simulink model "Appl_PaComfort_CtrlModel"  (R2018b)
settings: configuration reference "CodeConfig_10_ms" (kept outside this file)
undefined symbols (not defined in the file): D_CLOSE, D_InitDelayTime, D_OPEN, D_SoftDistancePaLegnth, D_WelcomeDistance, FALSE, TRUE
libraries: DareLib x44, simulink x1
(part 1 of 2)
settings Model: Creator=Administrator  LastModifiedBy=Administrator
settings ConfigSetRef: SourceLocation=Base Workspace

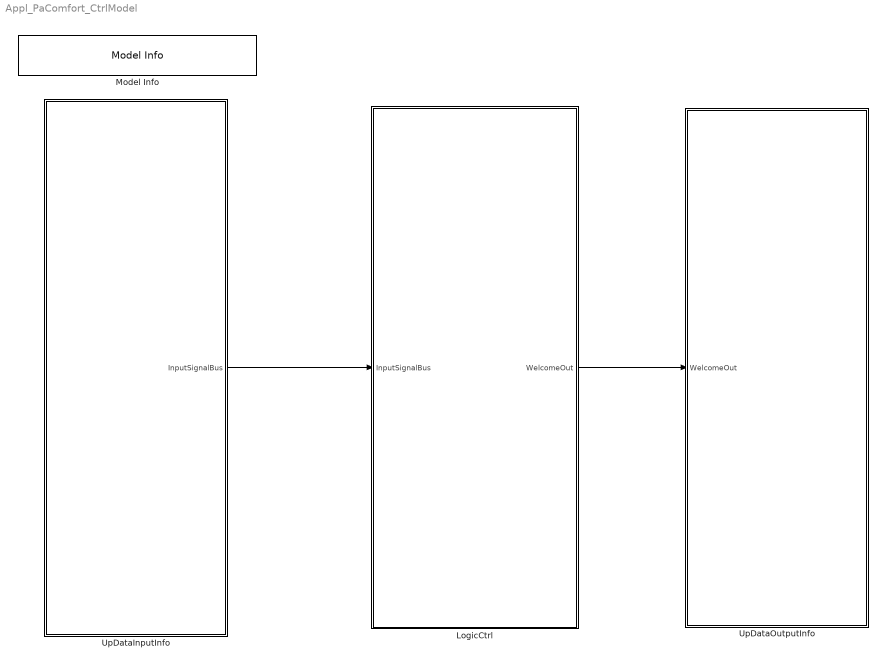
== system Appl_PaComfort_CtrlModel ==
  LogicCtrl : Subsystem  Priority=2  TreatAsAtomicUnit=on
      settings: RTWSystemCode=Nonreusable function  RTWFcnNameOpts=Use subsystem name
  Model Info : simulink/Model-Wide Utilities/Model Info  Frame=on  DisplayStringWithTags=Version：%<ModelVersion>  HorizontalTextAlignment=Center  LeftAlignmentValue=0.5
  UpDataInputInfo : Subsystem  Priority=1  TreatAsAtomicUnit=on
      settings: RTWSystemCode=Nonreusable function  RTWFcnNameOpts=Use subsystem name
  UpDataOutputInfo : Subsystem  Priority=3  TreatAsAtomicUnit=on
      settings: RTWSystemCode=Nonreusable function  RTWFcnNameOpts=Use subsystem name
  wires:
  LogicCtrl/1(WelcomeOut) -> UpDataOutputInfo/1(WelcomeOut)
  UpDataInputInfo/1(InputSignalBus) -> LogicCtrl/1(InputSignalBus)

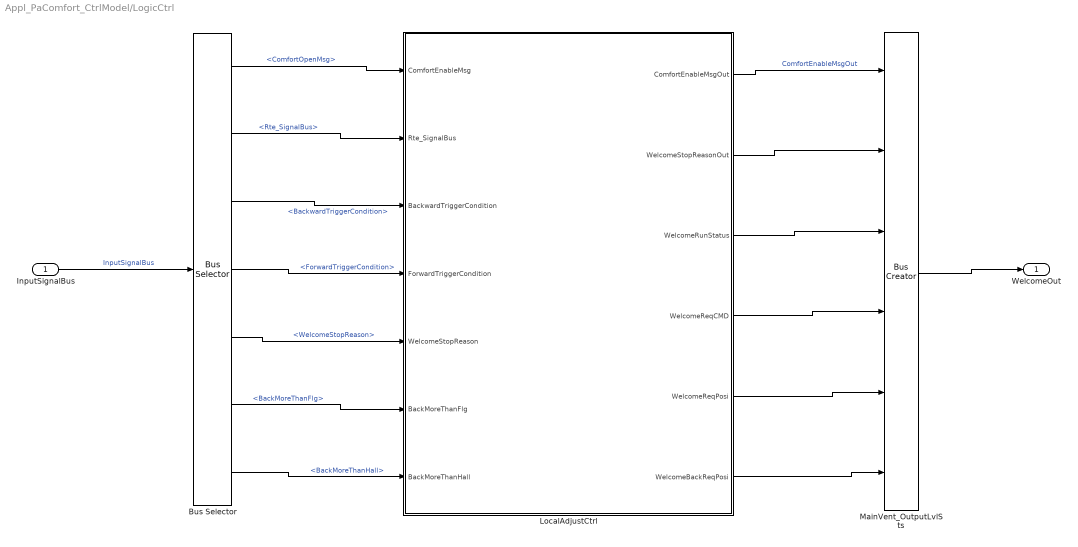
== system Appl_PaComfort_CtrlModel/LogicCtrl ==
  InputSignalBus : Inport
  Bus Selector : BusSelector  OutputSignals=ComfortOpenMsg,Rte_SignalBus,BackwardTriggerCondition,ForwardTriggerCondition,WelcomeStopReason,BackMoreThanFlg,BackMoreThanHall
  LocalAdjustCtrl : Subsystem  Description=加热逻辑处理
      settings: AttributesFormatString=%<Description>
  MainVent_OutputLvlSts : BusCreator  Inputs=6
  WelcomeOut : Outport
  wires:
  InputSignalBus/1 -> Bus Selector/1  "InputSignalBus"
  MainVent_OutputLvlSts/1 -> WelcomeOut/1
  Bus Selector/2 -> LocalAdjustCtrl/2(Rte_SignalBus)  "<Rte_SignalBus>"
  Bus Selector/3 -> LocalAdjustCtrl/3(BackwardTriggerCondition)  "<BackwardTriggerCondition>"
  Bus Selector/4 -> LocalAdjustCtrl/4(ForwardTriggerCondition)  "<ForwardTriggerCondition>"
  Bus Selector/5 -> LocalAdjustCtrl/5(WelcomeStopReason)  "<WelcomeStopReason>"
  Bus Selector/1 -> LocalAdjustCtrl/1(ComfortEnableMsg)  "<ComfortOpenMsg>"
  LocalAdjustCtrl/1(ComfortEnableMsgOut) -> MainVent_OutputLvlSts/1  "ComfortEnableMsgOut"
  LocalAdjustCtrl/2(WelcomeStopReasonOut) -> MainVent_OutputLvlSts/2
  LocalAdjustCtrl/3(WelcomeRunStatus) -> MainVent_OutputLvlSts/3
  LocalAdjustCtrl/4(WelcomeReqCMD) -> MainVent_OutputLvlSts/4
  LocalAdjustCtrl/5(WelcomeReqPosi) -> MainVent_OutputLvlSts/5
  Bus Selector/6 -> LocalAdjustCtrl/6(BackMoreThanFlg)  "<BackMoreThanFlg>"
  Bus Selector/7 -> LocalAdjustCtrl/7(BackMoreThanHall)  "<BackMoreThanHall>"
  LocalAdjustCtrl/6(WelcomeBackReqPosi) -> MainVent_OutputLvlSts/6

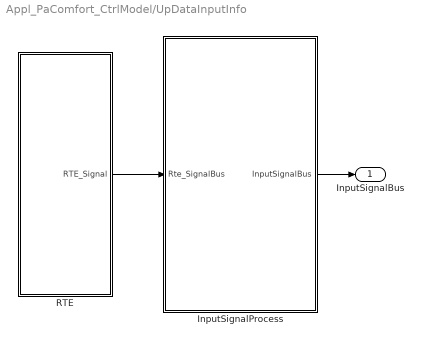
== system Appl_PaComfort_CtrlModel/UpDataInputInfo ==
  InputSignalProcess : Subsystem  Description=数据处理
      settings: AttributesFormatString=%<Description>  RTWSystemCode=Nonreusable function  RTWFcnNameOpts=Use subsystem name
  RTE : Subsystem  Description=接口自动生成  TreatAsAtomicUnit=on
      settings: AttributesFormatString=%<Description>  RTWSystemCode=Nonreusable function  RTWFcnNameOpts=Use subsystem name
  InputSignalBus : Outport
  wires:
  RTE/1(RTE_Signal) -> InputSignalProcess/1(Rte_SignalBus)
  InputSignalProcess/1(InputSignalBus) -> InputSignalBus/1

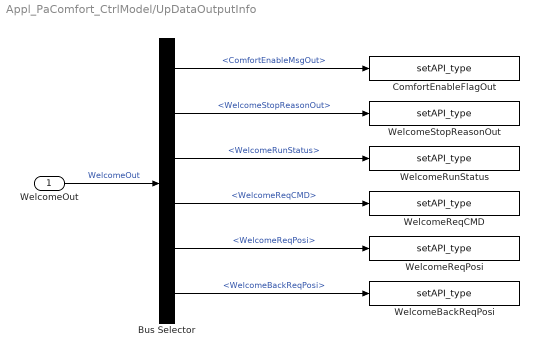
== system Appl_PaComfort_CtrlModel/UpDataOutputInfo ==
  WelcomeOut : Inport
  Bus Selector : BusSelector  OutputSignals=ComfortEnableMsgOut,WelcomeStopReasonOut,WelcomeRunStatus,WelcomeReqCMD,WelcomeReqPosi,WelcomeBackReqPosi
  ComfortEnableFlagOut : DareLib/Dare/setAPI_type  g_funcname=CanTx_0x3B2_DSM_St_FRSeatmeet  g_param=""  g_type=uint8  g_size=-1
      settings: AttributesFormatString=%<g_funcname>  SourceProductName=Dare Library
  WelcomeBackReqPosi : DareLib/Dare/setAPI_type  g_funcname=Rte_SetVfb_PaWelBackReqPosi  g_param=""  g_type=uint16  g_size=-1
      settings: AttributesFormatString=%<g_funcname>  SourceProductName=Dare Library
  WelcomeReqCMD : DareLib/Dare/setAPI_type  g_funcname=Rte_SetVfb_PaWelLengthReqCMD  g_param=""  g_type=uint8  g_size=-1
      settings: AttributesFormatString=%<g_funcname>  SourceProductName=Dare Library
  WelcomeReqPosi : DareLib/Dare/setAPI_type  g_funcname=Rte_SetVfb_PaWelLengthReqPosi  g_param=""  g_type=uint16  g_size=-1
      settings: AttributesFormatString=%<g_funcname>  SourceProductName=Dare Library
  WelcomeRunStatus : DareLib/Dare/setAPI_type  g_funcname=Rte_SetVfb_PaWelcomeRunSts  g_param=""  g_type=uint8  g_size=-1
      settings: AttributesFormatString=%<g_funcname>  SourceProductName=Dare Library
  WelcomeStopReasonOut : DareLib/Dare/setAPI_type  g_funcname=Rte_SetVfb_PaWelcomeStopReason  g_param=""  g_type=uint8  g_size=-1
      settings: AttributesFormatString=%<g_funcname>  SourceProductName=Dare Library
  wires:
  WelcomeOut/1 -> Bus Selector/1  "WelcomeOut"
  Bus Selector/4 -> WelcomeReqCMD/1  "<WelcomeReqCMD>"
  Bus Selector/3 -> WelcomeRunStatus/1  "<WelcomeRunStatus>"
  Bus Selector/2 -> WelcomeStopReasonOut/1  "<WelcomeStopReasonOut>"
  Bus Selector/1 -> ComfortEnableFlagOut/1  "<ComfortEnableMsgOut>"
  Bus Selector/5 -> WelcomeReqPosi/1  "<WelcomeReqPosi>"
  Bus Selector/6 -> WelcomeBackReqPosi/1  "<WelcomeBackReqPosi>"

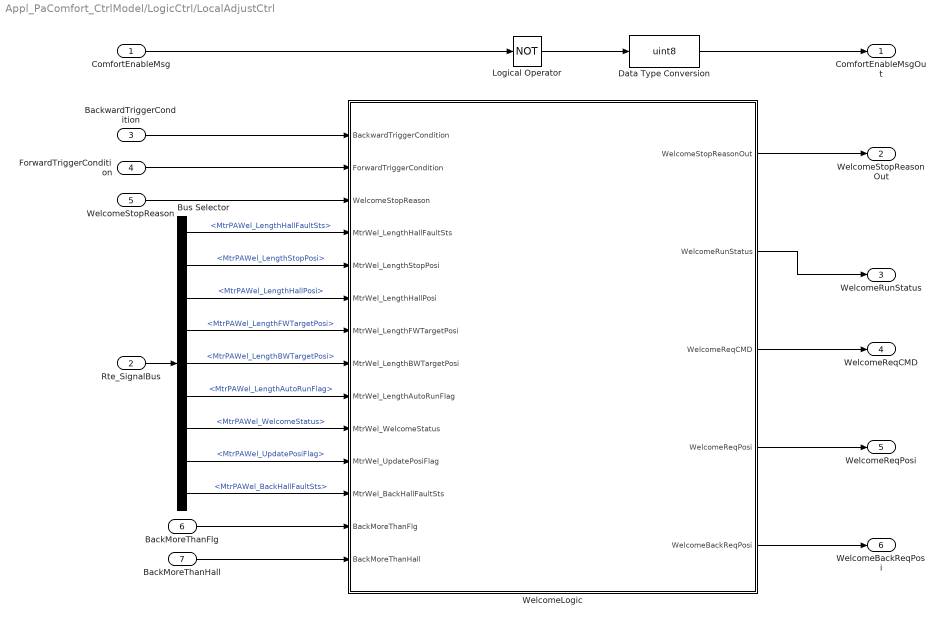
== system Appl_PaComfort_CtrlModel/LogicCtrl/LocalAdjustCtrl ==
  ComfortEnableMsg : Inport
  Rte_SignalBus : Inport  Port=2
  BackwardTriggerCondition : Inport  Port=3
  ForwardTriggerCondition : Inport  Port=4
  WelcomeStopReason : Inport  Port=5
  BackMoreThanFlg : Inport  Port=6
  BackMoreThanHall : Inport  Port=7
  Bus Selector : BusSelector  OutputSignals=MtrPAWel_LengthHallFaultSts,MtrPAWel_LengthStopPosi,MtrPAWel_LengthHallPosi,MtrPAWel_LengthFWTargetPosi,MtrPAWel_LengthBWTargetPosi,MtrPAWel_LengthAutoRunFlag,MtrPAWel_WelcomeStatus,MtrPAWel_UpdatePosiFlag,MtrPAWel_BackHallFaultSts
  Data Type Conversion : DataTypeConversion  OutDataTypeStr=uint8
  Logical Operator : Logic  Operator=NOT  AllPortsSameDT=off  OutDataTypeStr=boolean
  WelcomeLogic : Stateflow chart  TreatAsAtomicUnit=on
  ComfortEnableMsgOut : Outport
  WelcomeStopReasonOut : Outport  Port=2
  WelcomeRunStatus : Outport  Port=3
  WelcomeReqCMD : Outport  Port=4
  WelcomeReqPosi : Outport  Port=5
  WelcomeBackReqPosi : Outport  Port=6
  wires:
  ComfortEnableMsg/1 -> Logical Operator/1
  Rte_SignalBus/1 -> Bus Selector/1
  BackwardTriggerCondition/1 -> WelcomeLogic/1(BackwardTriggerCondition)
  ForwardTriggerCondition/1 -> WelcomeLogic/2(ForwardTriggerCondition)
  WelcomeStopReason/1 -> WelcomeLogic/3(WelcomeStopReason)
  Bus Selector/2 -> WelcomeLogic/5(MtrWel_LengthStopPosi)  "<MtrPAWel_LengthStopPosi>"
  Bus Selector/3 -> WelcomeLogic/6(MtrWel_LengthHallPosi)  "<MtrPAWel_LengthHallPosi>"
  Bus Selector/6 -> WelcomeLogic/9(MtrWel_LengthAutoRunFlag)  "<MtrPAWel_LengthAutoRunFlag>"
  Bus Selector/4 -> WelcomeLogic/7(MtrWel_LengthFWTargetPosi)  "<MtrPAWel_LengthFWTargetPosi>"
  Bus Selector/5 -> WelcomeLogic/8(MtrWel_LengthBWTargetPosi)  "<MtrPAWel_LengthBWTargetPosi>"
  Bus Selector/7 -> WelcomeLogic/10(MtrWel_WelcomeStatus)  "<MtrPAWel_WelcomeStatus>"
  WelcomeLogic/1(WelcomeStopReasonOut) -> WelcomeStopReasonOut/1
  WelcomeLogic/2(WelcomeRunStatus) -> WelcomeRunStatus/1
  WelcomeLogic/3(WelcomeReqCMD) -> WelcomeReqCMD/1
  WelcomeLogic/4(WelcomeReqPosi) -> WelcomeReqPosi/1
  Logical Operator/1 -> Data Type Conversion/1
  Data Type Conversion/1 -> ComfortEnableMsgOut/1
  Bus Selector/1 -> WelcomeLogic/4(MtrWel_LengthHallFaultSts)  "<MtrPAWel_LengthHallFaultSts>"
  Bus Selector/8 -> WelcomeLogic/11(MtrWel_UpdatePosiFlag)  "<MtrPAWel_UpdatePosiFlag>"
  BackMoreThanFlg/1 -> WelcomeLogic/13(BackMoreThanFlg)
  BackMoreThanHall/1 -> WelcomeLogic/14(BackMoreThanHall)
  Bus Selector/9 -> WelcomeLogic/12(MtrWel_BackHallFaultSts)  "<MtrPAWel_BackHallFaultSts>"
  WelcomeLogic/5(WelcomeBackReqPosi) -> WelcomeBackReqPosi/1

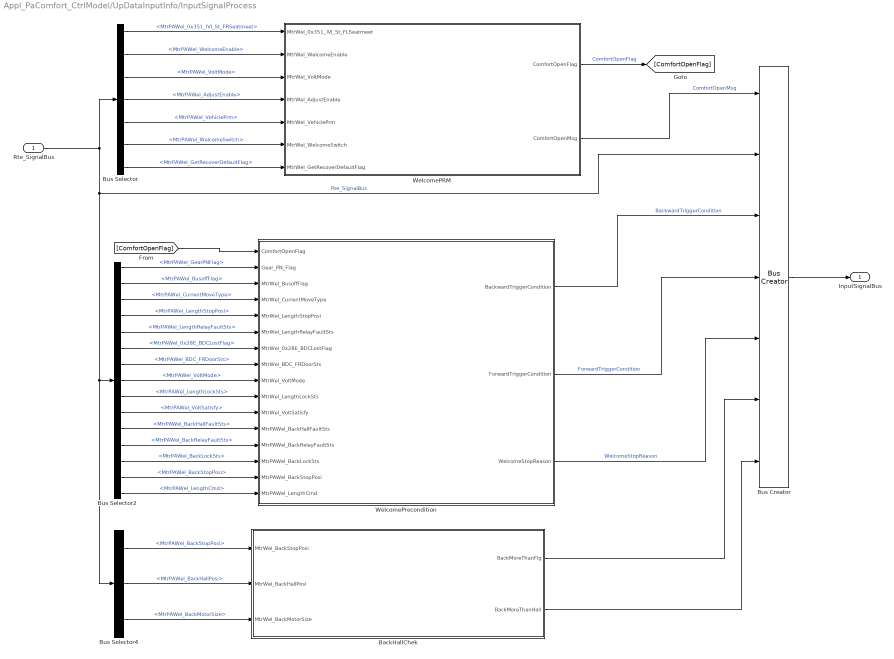
== system Appl_PaComfort_CtrlModel/UpDataInputInfo/InputSignalProcess ==
  Rte_SignalBus : Inport
  "BackHallChek " : Subsystem
  Bus Creator : BusCreator  Inputs=7
  Bus Selector : BusSelector  OutputSignals=MtrPAWel_0x351_IVI_St_FRSeatmeet,MtrPAWel_WelcomeEnable,MtrPAWel_VoltMode,MtrPAWel_AdjustEnable,MtrPAWel_VehiclePrm,MtrPAWel_WelcomeSwitch,MtrPAWel_GetRecoverDefaultFlag
  Bus Selector2 : BusSelector  OutputSignals=MtrPAWel_GearPNFlag,MtrPAWel_BusoffFlag,MtrPAWel_CurrentMoveType,MtrPAWel_LengthStopPosi,MtrPAWel_LengthRelayFaultSts,MtrPAWel_0x28E_BDCLostFlag,MtrPAWel_BDC_FRDoorSts,MtrPAWel_VoltMode,MtrPAWel_LengthLockSts,MtrPAWel_VoltSatisfy,MtrPAWel_BackHallFaultSts,MtrPAWel_BackRelayFaultSts,MtrPAWel_BackLockSts,MtrPAWel_BackStopPosi,MtrPAWel_LengthCmd
  Bus Selector4 : BusSelector  OutputSignals=MtrPAWel_BackStopPosi,MtrPAWel_BackHallPosi,MtrPAWel_BackMotorSize
  WelcomePRM : Subsystem  Description=迎宾配置
      settings: AttributesFormatString=%<Description>
  WelcomePrecondition : Subsystem  Description=迎宾前置条件
      settings: AttributesFormatString=%<Description>
  InputSignalBus : Outport
  wires:
  Bus Creator/1 -> InputSignalBus/1
  Rte_SignalBus/1 -> Bus Selector4/1, Bus Selector2/1, Bus Creator/2, Bus Selector/1  "Rte_SignalBus"
  WelcomePRM/1(ComfortOpenFlag) -> [ComfortOpenFlag]  "ComfortOpenFlag"
  Bus Selector/1 -> WelcomePRM/1(MtrWel_0x351_IVI_St_FLSeatmeet)  "<MtrPAWel_0x351_IVI_St_FRSeatmeet>"
  Bus Selector/3 -> WelcomePRM/3(MtrWel_VoltMode)  "<MtrPAWel_VoltMode>"
  WelcomePrecondition/1(BackwardTriggerCondition) -> Bus Creator/3  "BackwardTriggerCondition"
  WelcomePrecondition/2(ForwardTriggerCondition) -> Bus Creator/4  "ForwardTriggerCondition"
  WelcomePrecondition/3(WelcomeStopReason) -> Bus Creator/5  "WelcomeStopReason"
  Bus Selector/5 -> WelcomePRM/5(MtrWel_VehiclePrm)  "<MtrPAWel_VehiclePrm>"
  Bus Selector/6 -> WelcomePRM/6(MtrWel_WelcomeSwitch)  "<MtrPAWel_WelcomeSwitch>"
  Bus Selector/7 -> WelcomePRM/7(MtrWel_GetRecoverDefaultFlag)  "<MtrPAWel_GetRecoverDefaultFlag>"
  WelcomePRM/2(ComfortOpenMsg) -> Bus Creator/1  "ComfortOpenMsg"
  Bus Selector/2 -> WelcomePRM/2(MtrWel_WelcomeEnable)  "<MtrPAWel_WelcomeEnable>"
  Bus Selector/4 -> WelcomePRM/4(MtrWel_AdjustEnable)  "<MtrPAWel_AdjustEnable>"
  Bus Selector4/1 -> "BackHallChek "/1(MtrWel_BackStopPosi)  "<MtrPAWel_BackStopPosi>"
  Bus Selector4/2 -> "BackHallChek "/2(MtrWel_BackHallPosi)  "<MtrPAWel_BackHallPosi>"
  Bus Selector4/3 -> "BackHallChek "/3(MtrWel_BackMotorSize)  "<MtrPAWel_BackMotorSize>"
  "BackHallChek "/1(BackMoreThanFlg) -> Bus Creator/6
  "BackHallChek "/2(BackMoreThanHall) -> Bus Creator/7
  [ComfortOpenFlag] -> WelcomePrecondition/1(ComfortOpenFlag)
  Bus Selector2/1 -> WelcomePrecondition/2(Gear_PN_Flag)  "<MtrPAWel_GearPNFlag>"
  Bus Selector2/2 -> WelcomePrecondition/3(MtrWel_BusoffFlag)  "<MtrPAWel_BusoffFlag>"
  Bus Selector2/3 -> WelcomePrecondition/4(MtrWel_CurrentMoveType)  "<MtrPAWel_CurrentMoveType>"
  Bus Selector2/4 -> WelcomePrecondition/5(MtrWel_LengthStopPosi)  "<MtrPAWel_LengthStopPosi>"
  Bus Selector2/5 -> WelcomePrecondition/6(MtrWel_LengthRelayFaultSts)  "<MtrPAWel_LengthRelayFaultSts>"
  Bus Selector2/6 -> WelcomePrecondition/7(MtrWel_0x28E_BDCLostFlag)  "<MtrPAWel_0x28E_BDCLostFlag>"
  Bus Selector2/7 -> WelcomePrecondition/8(MtrWel_BDC_FRDoorSts)  "<MtrPAWel_BDC_FRDoorSts>"
  Bus Selector2/8 -> WelcomePrecondition/9(MtrWel_VoltMode)  "<MtrPAWel_VoltMode>"
  Bus Selector2/9 -> WelcomePrecondition/10(MtrWel_LengthLockSts)  "<MtrPAWel_LengthLockSts>"
  Bus Selector2/10 -> WelcomePrecondition/11(MtrWel_VoltSatisfy)  "<MtrPAWel_VoltSatisfy>"
  Bus Selector2/11 -> WelcomePrecondition/12(MtrPAWel_BackHallFaultSts)  "<MtrPAWel_BackHallFaultSts>"
  Bus Selector2/12 -> WelcomePrecondition/13(MtrPAWel_BackRelayFaultSts)  "<MtrPAWel_BackRelayFaultSts>"
  Bus Selector2/13 -> WelcomePrecondition/14(MtrPAWel_BackLockSts)  "<MtrPAWel_BackLockSts>"
  Bus Selector2/14 -> WelcomePrecondition/15(MtrPAWel_BackStopPosi)  "<MtrPAWel_BackStopPosi>"
  Bus Selector2/15 -> WelcomePrecondition/16(MtrPAWel_LengthCmd)  "<MtrPAWel_LengthCmd>"

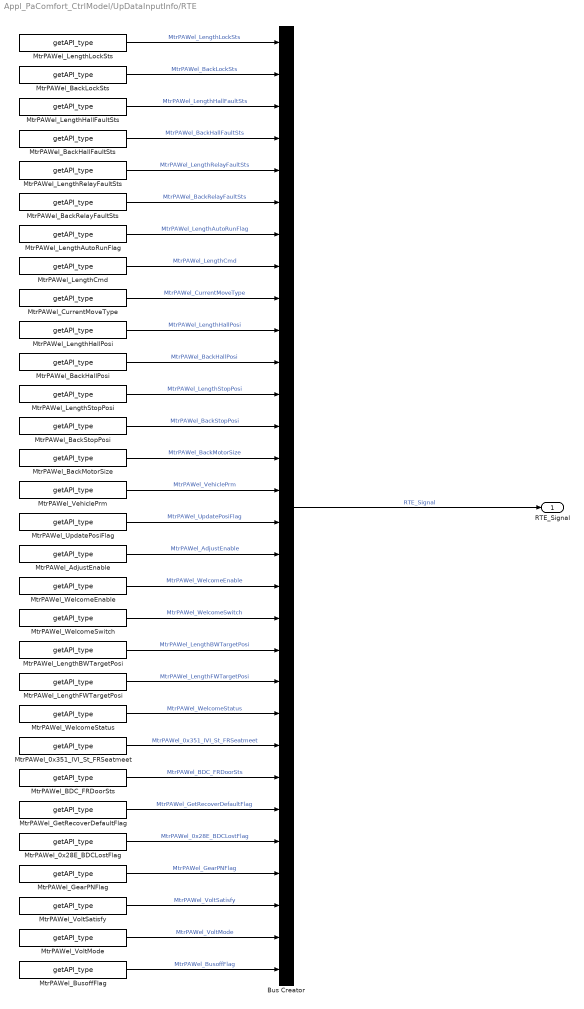
== system Appl_PaComfort_CtrlModel/UpDataInputInfo/RTE ==
  Bus Creator : BusCreator  Inputs=30
  MtrPAWel_0x28E_BDCLostFlag : DareLib/Dare/getAPI_type  g_funcname=Ecual_GetCanMsgLostFlag  g_param=eRXINDEX_0x28E  g_type=uint8  g_size=-1
      settings: AttributesFormatString=%<g_funcname>  SourceProductName=Dare Library
  MtrPAWel_0x351_IVI_St_FRSeatmeet : DareLib/Dare/getAPI_type  g_funcname=CanRx_0x351_IVI_St_FRSeatmeet  g_param=""  g_type=uint8  g_size=-1
      settings: AttributesFormatString=%<g_funcname>  SourceProductName=Dare Library
  MtrPAWel_AdjustEnable : DareLib/Dare/getAPI_type  g_funcname=Srvl_GetMemIndexDataU8  g_param=EN_MemIndex_PaAdjustConfig  g_type=uint8  g_size=-1
      settings: AttributesFormatString=%<g_funcname>  SourceProductName=Dare Library
  MtrPAWel_BDC_FRDoorSts : DareLib/Dare/getAPI_type  g_funcname=CanRx_0x28E_BDC_FRDoorSts  g_param=""  g_type=uint8  g_size=-1
      settings: AttributesFormatString=%<g_funcname>  SourceProductName=Dare Library
  MtrPAWel_BackHallFaultSts : DareLib/Dare/getAPI_type  g_funcname=Rte_GetVfb_PaBackHallErr  g_param=""  g_type=uint8  g_size=-1
      settings: AttributesFormatString=%<g_funcname>  SourceProductName=Dare Library
  MtrPAWel_BackHallPosi : DareLib/Dare/getAPI_type  g_funcname=Cdd_GetCurrentHallCnt  g_param=EN_PassengerBack  g_type=uint16  g_size=-1
      settings: AttributesFormatString=%<g_funcname>  SourceProductName=Dare Library
  MtrPAWel_BackLockSts : DareLib/Dare/getAPI_type  g_funcname=Rte_GetVfb_PaBackStallErr  g_param=""  g_type=uint8  g_size=-1
      settings: AttributesFormatString=%<g_funcname>  SourceProductName=Dare Library
  MtrPAWel_BackMotorSize : DareLib/Dare/getAPI_type  g_funcname=Cdd_GetMotorSize  g_param=EN_PassengerBack  g_type=uint16  g_size=-1
      settings: AttributesFormatString=%<g_funcname>  SourceProductName=Dare Library
  MtrPAWel_BackRelayFaultSts : DareLib/Dare/getAPI_type  g_funcname=Rte_GetVfb_PaBackRelayAdheErr  g_param=""  g_type=uint8  g_size=-1
      settings: AttributesFormatString=%<g_funcname>  SourceProductName=Dare Library
  MtrPAWel_BackStopPosi : DareLib/Dare/getAPI_type  g_funcname=Cdd_GetMotorHardStop  g_param=EN_PassengerBack  g_type=uint16  g_size=-1
      settings: AttributesFormatString=%<g_funcname>  SourceProductName=Dare Library
  MtrPAWel_BusoffFlag : DareLib/Dare/getAPI_type  g_funcname=Nm_IsBusOff  g_param=""  g_type=uint8  g_size=-1
      settings: AttributesFormatString=%<g_funcname>  SourceProductName=Dare Library
  MtrPAWel_CurrentMoveType : DareLib/Dare/getAPI_type  g_funcname=Rte_GetVfb_PaMoveType  g_param=""  g_type=uint8  g_enum=enSeatMotorRunType  g_size=-1
      settings: AttributesFormatString=%<g_funcname>  SourceProductName=Dare Library
  MtrPAWel_GearPNFlag : DareLib/Dare/getAPI_type  g_funcname=Rte_GetCAN_Gear_PN_Flag  g_param=""  g_type=uint8  g_size=-1
      settings: AttributesFormatString=%<g_funcname>  SourceProductName=Dare Library
  MtrPAWel_GetRecoverDefaultFlag : DareLib/Dare/getAPI_type  g_funcname=GetRecoverDefaultFlag  g_param=""  g_type=uint8  g_size=-1
      settings: AttributesFormatString=%<g_funcname>  SourceProductName=Dare Library
  MtrPAWel_LengthAutoRunFlag : DareLib/Dare/getAPI_type  g_funcname=Rte_GetVfb_PaLengthAutoRunFlag  g_param=""  g_type=uint8  g_enum=enSeatAutoRunSts  g_size=-1
      settings: AttributesFormatString=%<g_funcname>  SourceProductName=Dare Library
  MtrPAWel_LengthBWTargetPosi : DareLib/Dare/getAPI_type  g_funcname=Srvl_GetMemIndexDataU16  g_param=EN_MemIndex_PaWelcome_LenTar_BackWard  g_type=uint16  g_size=-1
      settings: AttributesFormatString=%<g_funcname>  SourceProductName=Dare Library
  MtrPAWel_LengthCmd : DareLib/Dare/getAPI_type  g_funcname=Rte_GetVfb_PaLengthMotorCmd  g_param=""  g_type=uint8  g_size=-1
      settings: AttributesFormatString=%<g_funcname>  SourceProductName=Dare Library
  MtrPAWel_LengthFWTargetPosi : DareLib/Dare/getAPI_type  g_funcname=Srvl_GetMemIndexDataU16  g_param=EN_MemIndex_PaWelcome_LenTar_ForWard  g_type=uint16  g_size=-1
      settings: AttributesFormatString=%<g_funcname>  SourceProductName=Dare Library
  MtrPAWel_LengthHallFaultSts : DareLib/Dare/getAPI_type  g_funcname=Rte_GetVfb_PaLengthHallErr  g_param=""  g_type=uint8  g_size=-1
      settings: AttributesFormatString=%<g_funcname>  SourceProductName=Dare Library
  MtrPAWel_LengthHallPosi : DareLib/Dare/getAPI_type  g_funcname=Cdd_GetCurrentHallCnt  g_param=EN_PassengerLength  g_type=uint16  g_size=-1
      settings: AttributesFormatString=%<g_funcname>  SourceProductName=Dare Library
  MtrPAWel_LengthLockSts : DareLib/Dare/getAPI_type  g_funcname=Rte_GetVfb_PaLengthStallErr  g_param=""  g_type=uint8  g_size=-1
      settings: AttributesFormatString=%<g_funcname>  SourceProductName=Dare Library
  MtrPAWel_LengthRelayFaultSts : DareLib/Dare/getAPI_type  g_funcname=Rte_GetVfb_PaLengthRelayAdheErr  g_param=""  g_type=uint8  g_size=-1
      settings: AttributesFormatString=%<g_funcname>  SourceProductName=Dare Library
  MtrPAWel_LengthStopPosi : DareLib/Dare/getAPI_type  g_funcname=Cdd_GetMotorHardStop  g_param=EN_PassengerLength  g_type=uint16  g_size=-1
      settings: AttributesFormatString=%<g_funcname>  SourceProductName=Dare Library
  MtrPAWel_UpdatePosiFlag : DareLib/Dare/getAPI_type  g_funcname=Srvl_GetMemIndexDataU8  g_param=EN_MemIndex_WelcomePaUpdate  g_type=uint8  g_size=-1
      settings: AttributesFormatString=%<g_funcname>  SourceProductName=Dare Library
  MtrPAWel_VehiclePrm : DareLib/Dare/getAPI_type  g_funcname=Srvl_GetMemIndexDataU8  g_param=EN_MemIndex_Heat_CarType  g_type=uint8  g_enum=enVehTypePrm  g_size=-1
      settings: AttributesFormatString=%<g_funcname>  SourceProductName=Dare Library
  MtrPAWel_VoltMode : DareLib/Dare/getAPI_type  g_funcname=Rte_GetVfb_VoltMode  g_param=""  g_type=uint8  g_enum=enFinalPowerMode  g_size=-1
      settings: AttributesFormatString=%<g_funcname>  SourceProductName=Dare Library
  MtrPAWel_VoltSatisfy : DareLib/Dare/getAPI_type  g_funcname=Rte_GetVfb_VoltSatisfy  g_param=""  g_type=uint8  g_size=-1
      settings: AttributesFormatString=%<g_funcname>  SourceProductName=Dare Library
  MtrPAWel_WelcomeEnable : DareLib/Dare/getAPI_type  g_funcname=Srvl_GetMemIndexDataU8  g_param=EN_MemIndex_PaMemoryConfig  g_type=uint8  g_size=-1
      settings: AttributesFormatString=%<g_funcname>  SourceProductName=Dare Library
  MtrPAWel_WelcomeStatus : DareLib/Dare/getAPI_type  g_funcname=Srvl_GetMemIndexDataU8  g_param=EN_MemIndex_PaWelcomeStatus  g_type=uint8  g_enum=enWelcomeSts  g_size=-1
      settings: AttributesFormatString=%<g_funcname>  SourceProductName=Dare Library
  MtrPAWel_WelcomeSwitch : DareLib/Dare/getAPI_type  g_funcname=Srvl_GetMemIndexDataU8  g_param=EN_MemIndex_PaWelcomeSwitch  g_type=uint8  g_size=-1
      settings: AttributesFormatString=%<g_funcname>  SourceProductName=Dare Library
  RTE_Signal : Outport
  wires:
  Bus Creator/1 -> RTE_Signal/1  "RTE_Signal"
  MtrPAWel_LengthLockSts/1 -> Bus Creator/1  "MtrPAWel_LengthLockSts"
  MtrPAWel_BackLockSts/1 -> Bus Creator/2  "MtrPAWel_BackLockSts"
  MtrPAWel_LengthHallFaultSts/1 -> Bus Creator/3  "MtrPAWel_LengthHallFaultSts"
  MtrPAWel_BackHallFaultSts/1 -> Bus Creator/4  "MtrPAWel_BackHallFaultSts"
  MtrPAWel_LengthRelayFaultSts/1 -> Bus Creator/5  "MtrPAWel_LengthRelayFaultSts"
  MtrPAWel_BackRelayFaultSts/1 -> Bus Creator/6  "MtrPAWel_BackRelayFaultSts"
  MtrPAWel_LengthAutoRunFlag/1 -> Bus Creator/7  "MtrPAWel_LengthAutoRunFlag"
  MtrPAWel_LengthCmd/1 -> Bus Creator/8  "MtrPAWel_LengthCmd"
  MtrPAWel_CurrentMoveType/1 -> Bus Creator/9  "MtrPAWel_CurrentMoveType"
  MtrPAWel_LengthHallPosi/1 -> Bus Creator/10  "MtrPAWel_LengthHallPosi"
  MtrPAWel_BackHallPosi/1 -> Bus Creator/11  "MtrPAWel_BackHallPosi"
  MtrPAWel_LengthStopPosi/1 -> Bus Creator/12  "MtrPAWel_LengthStopPosi"
  MtrPAWel_BackStopPosi/1 -> Bus Creator/13  "MtrPAWel_BackStopPosi"
  MtrPAWel_BackMotorSize/1 -> Bus Creator/14  "MtrPAWel_BackMotorSize"
  MtrPAWel_VehiclePrm/1 -> Bus Creator/15  "MtrPAWel_VehiclePrm"
  MtrPAWel_UpdatePosiFlag/1 -> Bus Creator/16  "MtrPAWel_UpdatePosiFlag"
  MtrPAWel_AdjustEnable/1 -> Bus Creator/17  "MtrPAWel_AdjustEnable"
  MtrPAWel_WelcomeEnable/1 -> Bus Creator/18  "MtrPAWel_WelcomeEnable"
  MtrPAWel_WelcomeSwitch/1 -> Bus Creator/19  "MtrPAWel_WelcomeSwitch"
  MtrPAWel_LengthBWTargetPosi/1 -> Bus Creator/20  "MtrPAWel_LengthBWTargetPosi"
  MtrPAWel_LengthFWTargetPosi/1 -> Bus Creator/21  "MtrPAWel_LengthFWTargetPosi"
  MtrPAWel_WelcomeStatus/1 -> Bus Creator/22  "MtrPAWel_WelcomeStatus"
  MtrPAWel_0x351_IVI_St_FRSeatmeet/1 -> Bus Creator/23  "MtrPAWel_0x351_IVI_St_FRSeatmeet"
  MtrPAWel_BDC_FRDoorSts/1 -> Bus Creator/24  "MtrPAWel_BDC_FRDoorSts"
  MtrPAWel_GetRecoverDefaultFlag/1 -> Bus Creator/25  "MtrPAWel_GetRecoverDefaultFlag"
  MtrPAWel_0x28E_BDCLostFlag/1 -> Bus Creator/26  "MtrPAWel_0x28E_BDCLostFlag"
  MtrPAWel_GearPNFlag/1 -> Bus Creator/27  "MtrPAWel_GearPNFlag"
  MtrPAWel_VoltSatisfy/1 -> Bus Creator/28  "MtrPAWel_VoltSatisfy"
  MtrPAWel_VoltMode/1 -> Bus Creator/29  "MtrPAWel_VoltMode"
  MtrPAWel_BusoffFlag/1 -> Bus Creator/30  "MtrPAWel_BusoffFlag"

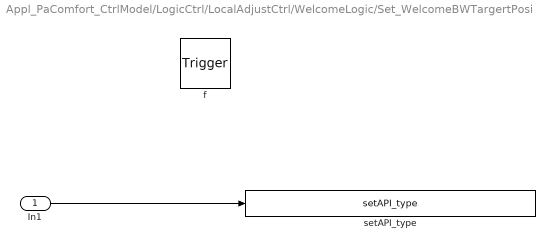
== system Appl_PaComfort_CtrlModel/LogicCtrl/LocalAdjustCtrl/WelcomeLogic/Set_WelcomeBWTargertPosi ==
  In1 : Inport
  f : TriggerPort  TriggerType=function-call  VariantControl=(inherit)
      settings: CopyFcn=Stateflow.SLINSF.SimulinkMan.removeBlockPreDeleteFcn  PreDeleteFcn=Stateflow.SLINSF.SimulinkMan.unsafePredeleteFcn
  setAPI_type : DareLib/Dare/setAPI_type  g_funcname=Srvl_SetMemIndexDataU16  g_param=EN_MemIndex_PaWelcome_LenTar_BackWard  g_type=uint16  g_size=-1
      settings: AttributesFormatString=%<g_funcname>  SourceProductName=Dare Library
  wires:
  In1/1 -> setAPI_type/1

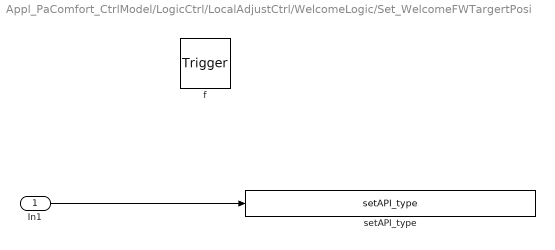
== system Appl_PaComfort_CtrlModel/LogicCtrl/LocalAdjustCtrl/WelcomeLogic/Set_WelcomeFWTargertPosi ==
  In1 : Inport
  f : TriggerPort  TriggerType=function-call  VariantControl=(inherit)
      settings: CopyFcn=Stateflow.SLINSF.SimulinkMan.removeBlockPreDeleteFcn  PreDeleteFcn=Stateflow.SLINSF.SimulinkMan.unsafePredeleteFcn
  setAPI_type : DareLib/Dare/setAPI_type  g_funcname=Srvl_SetMemIndexDataU16  g_param=EN_MemIndex_PaWelcome_LenTar_ForWard  g_type=uint16  g_size=-1
      settings: AttributesFormatString=%<g_funcname>  SourceProductName=Dare Library
  wires:
  In1/1 -> setAPI_type/1

== system Appl_PaComfort_CtrlModel/LogicCtrl/LocalAdjustCtrl/WelcomeLogic/Set_WelcomeStatus ==
  In1 : Inport
  f : TriggerPort  TriggerType=function-call  VariantControl=(inherit)
      settings: CopyFcn=Stateflow.SLINSF.SimulinkMan.removeBlockPreDeleteFcn  PreDeleteFcn=Stateflow.SLINSF.SimulinkMan.unsafePredeleteFcn
  setAPI_type : DareLib/Dare/setAPI_type  g_funcname=Srvl_SetMemIndexDataU8  g_param=EN_MemIndex_PaWelcomeStatus  g_type=uint8  g_size=-1
      settings: AttributesFormatString=%<g_funcname>  SourceProductName=Dare Library
  wires:
  In1/1 -> setAPI_type/1

== system Appl_PaComfort_CtrlModel/LogicCtrl/LocalAdjustCtrl/WelcomeLogic/Set_WelcomeUpdatePosiFlag ==
  In1 : Inport
  f : TriggerPort  TriggerType=function-call  VariantControl=(inherit)
      settings: CopyFcn=Stateflow.SLINSF.SimulinkMan.removeBlockPreDeleteFcn  PreDeleteFcn=Stateflow.SLINSF.SimulinkMan.unsafePredeleteFcn
  setAPI_type : DareLib/Dare/setAPI_type  g_funcname=Srvl_SetMemIndexDataU8  g_param=EN_MemIndex_WelcomePaUpdate  g_type=uint16  g_size=-1
      settings: AttributesFormatString=%<g_funcname>  SourceProductName=Dare Library
  wires:
  In1/1 -> setAPI_type/1

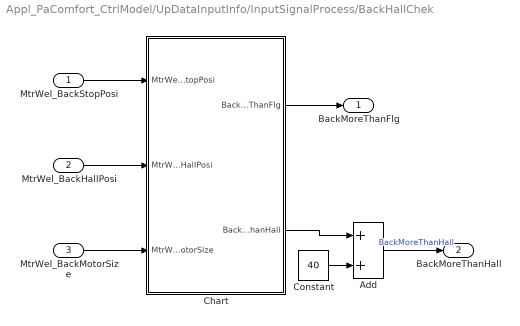
== system Appl_PaComfort_CtrlModel/UpDataInputInfo/InputSignalProcess/BackHallChek  ==
  MtrWel_BackStopPosi : Inport
  MtrWel_BackHallPosi : Inport  Port=2
  MtrWel_BackMotorSize : Inport  Port=3
  Add : Sum  AccumDataTypeStr=uint16
  Chart : Stateflow chart  TreatAsAtomicUnit=on
  Constant : Constant  Value=40  OutDataTypeStr=uint16
  BackMoreThanFlg : Outport
  BackMoreThanHall : Outport  Port=2
  wires:
  MtrWel_BackStopPosi/1 -> Chart/1(MtrWel_BackStopPosi)
  MtrWel_BackHallPosi/1 -> Chart/2(MtrWel_BackHallPosi)
  MtrWel_BackMotorSize/1 -> Chart/3(MtrWel_BackMotorSize)
  Chart/1(BackMoreThanFlg) -> BackMoreThanFlg/1
  Chart/2(BackMoreThanHall) -> Add/1
  Constant/1 -> Add/2
  Add/1 -> BackMoreThanHall/1  "BackMoreThanHall"

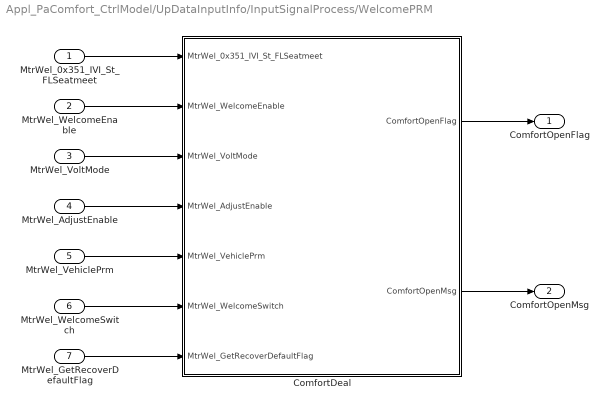
== system Appl_PaComfort_CtrlModel/UpDataInputInfo/InputSignalProcess/WelcomePRM ==
  MtrWel_0x351_IVI_St_FLSeatmeet : Inport
  MtrWel_WelcomeEnable : Inport  Port=2
  MtrWel_VoltMode : Inport  Port=3
  MtrWel_AdjustEnable : Inport  Port=4
  MtrWel_VehiclePrm : Inport  Port=5
  MtrWel_WelcomeSwitch : Inport  Port=6
  MtrWel_GetRecoverDefaultFlag : Inport  Port=7
  ComfortDeal : Stateflow chart  TreatAsAtomicUnit=on
  ComfortOpenFlag : Outport
  ComfortOpenMsg : Outport  Port=2
  wires:
  MtrWel_VoltMode/1 -> ComfortDeal/3(MtrWel_VoltMode)
  MtrWel_0x351_IVI_St_FLSeatmeet/1 -> ComfortDeal/1(MtrWel_0x351_IVI_St_FLSeatmeet)
  MtrWel_WelcomeEnable/1 -> ComfortDeal/2(MtrWel_WelcomeEnable)
  ComfortDeal/1(ComfortOpenFlag) -> ComfortOpenFlag/1
  MtrWel_AdjustEnable/1 -> ComfortDeal/4(MtrWel_AdjustEnable)
  MtrWel_VehiclePrm/1 -> ComfortDeal/5(MtrWel_VehiclePrm)
  MtrWel_WelcomeSwitch/1 -> ComfortDeal/6(MtrWel_WelcomeSwitch)
  MtrWel_GetRecoverDefaultFlag/1 -> ComfortDeal/7(MtrWel_GetRecoverDefaultFlag)
  ComfortDeal/2(ComfortOpenMsg) -> ComfortOpenMsg/1

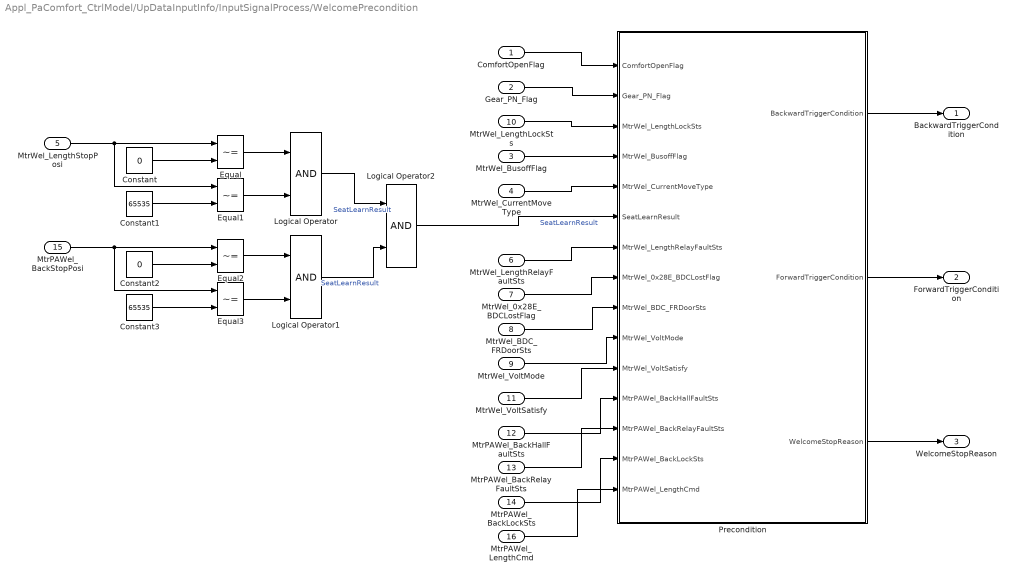
== system Appl_PaComfort_CtrlModel/UpDataInputInfo/InputSignalProcess/WelcomePrecondition ==
  ComfortOpenFlag : Inport
  Gear_PN_Flag : Inport  Port=2
  MtrWel_BusoffFlag : Inport  Port=3
  MtrWel_CurrentMoveType : Inport  Port=4
  MtrWel_LengthStopPosi : Inport  Port=5
  MtrWel_LengthRelayFaultSts : Inport  Port=6
  MtrWel_0x28E_BDCLostFlag : Inport  Port=7
  MtrWel_BDC_FRDoorSts : Inport  Port=8
  MtrWel_VoltMode : Inport  Port=9
  MtrWel_LengthLockSts : Inport  Port=10
  MtrWel_VoltSatisfy : Inport  Port=11
  MtrPAWel_BackHallFaultSts : Inport  Port=12
  MtrPAWel_BackRelayFaultSts : Inport  Port=13
  MtrPAWel_BackLockSts : Inport  Port=14
  MtrPAWel_BackStopPosi : Inport  Port=15
  MtrPAWel_LengthCmd : Inport  Port=16
  Constant : Constant  Value=0
  Constant1 : Constant  Value=65535
  Constant2 : Constant  Value=0
  Constant3 : Constant  Value=65535
  Equal{,1..3} (4 alike) : RelationalOperator  Operator=~=  OutDataTypeStr=boolean  RndMeth=Simplest
  Logical Operator : Logic  AllPortsSameDT=off  OutDataTypeStr=boolean
  Logical Operator1 : Logic  AllPortsSameDT=off  OutDataTypeStr=boolean
  Logical Operator2 : Logic  AllPortsSameDT=off  OutDataTypeStr=boolean
  Precondition : Stateflow chart  TreatAsAtomicUnit=on
  BackwardTriggerCondition : Outport
  ForwardTriggerCondition : Outport  Port=2
  WelcomeStopReason : Outport  Port=3
  wires:
  MtrWel_VoltSatisfy/1 -> Precondition/11(MtrWel_VoltSatisfy)
  MtrWel_BDC_FRDoorSts/1 -> Precondition/9(MtrWel_BDC_FRDoorSts)
  MtrWel_LengthStopPosi/1 -> Equal1/1, Equal/1
  Logical Operator/1 -> Logical Operator2/1  "SeatLearnResult"
  Constant1/1 -> Equal1/2
  MtrWel_0x28E_BDCLostFlag/1 -> Precondition/8(MtrWel_0x28E_BDCLostFlag)
  Equal/1 -> Logical Operator/1
  MtrWel_CurrentMoveType/1 -> Precondition/5(MtrWel_CurrentMoveType)
  MtrWel_VoltMode/1 -> Precondition/10(MtrWel_VoltMode)
  ComfortOpenFlag/1 -> Precondition/1(ComfortOpenFlag)
  MtrWel_LengthLockSts/1 -> Precondition/3(MtrWel_LengthLockSts)
  MtrWel_LengthRelayFaultSts/1 -> Precondition/7(MtrWel_LengthRelayFaultSts)
  Precondition/3(WelcomeStopReason) -> WelcomeStopReason/1
  MtrWel_BusoffFlag/1 -> Precondition/4(MtrWel_BusoffFlag)
  Gear_PN_Flag/1 -> Precondition/2(Gear_PN_Flag)
  Equal1/1 -> Logical Operator/2
  Precondition/2(ForwardTriggerCondition) -> ForwardTriggerCondition/1
  Constant/1 -> Equal/2
  Precondition/1(BackwardTriggerCondition) -> BackwardTriggerCondition/1
  MtrPAWel_BackLockSts/1 -> Precondition/14(MtrPAWel_BackLockSts)
  MtrPAWel_BackHallFaultSts/1 -> Precondition/12(MtrPAWel_BackHallFaultSts)
  MtrPAWel_BackRelayFaultSts/1 -> Precondition/13(MtrPAWel_BackRelayFaultSts)
  Constant2/1 -> Equal2/2
  Equal3/1 -> Logical Operator1/2
  Equal2/1 -> Logical Operator1/1
  Constant3/1 -> Equal3/2
  Logical Operator1/1 -> Logical Operator2/2  "SeatLearnResult"
  MtrPAWel_BackStopPosi/1 -> Equal3/1, Equal2/1
  Logical Operator2/1 -> Precondition/6(SeatLearnResult)  "SeatLearnResult"
  MtrPAWel_LengthCmd/1 -> Precondition/15(MtrPAWel_LengthCmd)

== system Appl_PaComfort_CtrlModel/UpDataInputInfo/InputSignalProcess/WelcomePRM/ComfortDeal/SetComfortPrm ==
  in : Inport
  f : TriggerPort  TriggerType=function-call  VariantControl=(inherit)
      settings: CopyFcn=Stateflow.SLINSF.SimulinkMan.removeBlockPreDeleteFcn  PreDeleteFcn=Stateflow.SLINSF.SimulinkMan.unsafePredeleteFcn
  setAPI_type : DareLib/Dare/setAPI_type  g_funcname=Srvl_SetMemIndexDataU8  g_param=EN_MemIndex_PaWelcomeSwitch  g_type=uint8  g_size=-1
      settings: AttributesFormatString=%<g_funcname>  SourceProductName=Dare Library
  wires:
  in/1 -> setAPI_type/1

== system Appl_PaComfort_CtrlModel/UpDataInputInfo/InputSignalProcess/WelcomePrecondition/Precondition/Get_DoorSts ==
  f : TriggerPort  TriggerType=function-call  VariantControl=(inherit)
      settings: CopyFcn=Stateflow.SLINSF.SimulinkMan.removeBlockPreDeleteFcn  PreDeleteFcn=Stateflow.SLINSF.SimulinkMan.unsafePredeleteFcn
  MtrWel_WelcomeSwitch : DareLib/Dare/getAPI_type  g_funcname=Srvl_GetMemIndexDataU8  g_param=EN_MemIndex_PaDoorSts  g_type=uint8  g_size=-1
      settings: AttributesFormatString=%<g_funcname>  SourceProductName=Dare Library
  Out1 : Outport
  wires:
  MtrWel_WelcomeSwitch/1 -> Out1/1

== system Appl_PaComfort_CtrlModel/UpDataInputInfo/InputSignalProcess/WelcomePrecondition/Precondition/Set_DoorSts ==
  In1 : Inport
  f : TriggerPort  TriggerType=function-call  VariantControl=(inherit)
      settings: CopyFcn=Stateflow.SLINSF.SimulinkMan.removeBlockPreDeleteFcn  PreDeleteFcn=Stateflow.SLINSF.SimulinkMan.unsafePredeleteFcn
  setAPI_type : DareLib/Dare/setAPI_type  g_funcname=Srvl_SetMemIndexDataU8  g_param=EN_MemIndex_PaDoorSts  g_type=uint8  g_size=-1
      settings: AttributesFormatString=%<g_funcname>  SourceProductName=Dare Library
  wires:
  In1/1 -> setAPI_type/1

== system Appl_PaComfort_CtrlModel/UpDataInputInfo/InputSignalProcess/WelcomePrecondition/Precondition/Set_WelcomeUpdatePosiFlag ==
  In1 : Inport
  f : TriggerPort  TriggerType=function-call  VariantControl=(inherit)
      settings: CopyFcn=Stateflow.SLINSF.SimulinkMan.removeBlockPreDeleteFcn  PreDeleteFcn=Stateflow.SLINSF.SimulinkMan.unsafePredeleteFcn
  setAPI_type : DareLib/Dare/setAPI_type  g_funcname=Srvl_SetMemIndexDataU8  g_param=EN_MemIndex_WelcomePaUpdate  g_type=uint16  g_size=-1
      settings: AttributesFormatString=%<g_funcname>  SourceProductName=Dare Library
  wires:
  In1/1 -> setAPI_type/1

== stateflow chart Appl_PaComfort_CtrlModel/UpDataInputInfo/InputSignalProcess/BackHallChek /Chart ==
  state Check [parallel]
    en:
    BackMoreThanHall = MtrWel_BackStopPosi + (MtrWel_BackMotorSize / 4);
    du:
    BackMoreThanHall = MtrWel_BackStopPosi + (MtrWel_BackMotorSize / 4);
    settings: executionOrder=1
  state More [parallel]
    settings: executionOrder=2
    state Init
      en:
      BackMoreThanFlg = FALSE;
    state MoreThan
      en:
      BackMoreThanFlg = TRUE;
    (default) -> Init
    Init -> MoreThan : /* 大于距前止点60°位置 */
        | [MtrWel_BackHallPosi > BackMoreThanHall]
    MoreThan -> Init : /* 小于等于距前止点60°位置 */
        | [MtrWel_BackHallPosi <= BackMoreThanHall]
  data: MtrWel_BackStopPosi input; MtrWel_BackHallPosi input; MtrWel_BackMotorSize input; BackMoreThanFlg output uint8; TRUE parameter; FALSE parameter; BackMoreThanHall output uint16

== stateflow chart Appl_PaComfort_CtrlModel/LogicCtrl/LocalAdjustCtrl/WelcomeLogic ==
  state WelcomeInactive
    en:
    /*更新停止原因、清空舒适请求、纵向坐标、更新迎宾状态*/
    /*迎宾未激活：1.舒适请求 = 无； 2.迎宾坐标 = 0；*/
    WelcomeReqCMD = FALSE;
    WelcomeReqPosi = 0;
    WelcomeBackReqPosi = 0;
    WelcomeFromeInitFlag = FALSE;
    WelcomeStatus = enWelcomeSts.EN_NULL;
    Set_WelcomeStatus(WelcomeStatus);
    WelcomeRunStatus = 10;
    WelcomeInactive -> (junction 307) [order 1]
    (default) -> (junction 307)
    (junction 307) -> (junction 308) [order 1] : /*如果输入禁能原因非空，则更新输出停止原因*/
        | [enWelStopCause.EN_WelStop_NULL != WelcomeStopReason]
    (junction 307) -> (junction 309) [order 2]
    (junction 308) -> (junction 311) : {WelcomeStopReasonOut = WelcomeStopReason;
        | WelcomeRunStatus = 12;
        | /*mantis：7341存在EEPORM存储失败*/
        | Set_WelcomeStatus(WelcomeStatus);}
    (junction 311) -> (junction 309)
    (junction 309) -> (junction 312)
  state Init
    en:
    InitTimer = 0;
    du:
    InitTimer++;
    ex:
    InitTimer = 0;
  state Set_WelcomeUpdatePosiFlag(In1) [function]
  state Set_WelcomeStatus(In1) [function]
  state Set_WelcomeBWTargertPosi(In1) [function]
  state Set_WelcomeFWTargertPosi(In1) [function]
  state WelcomeActive
    state WelcomeDefault
      en:
      /*迎宾默认状态：1.舒适请求 = 无； 2.迎宾坐标 = 0；*/
      WelcomeReqCMD = FALSE;
      WelcomeReqPosi = 0;
      WelcomeBackReqPosi = 0;
    state WelcomeBackward
      state BackCheck
        (default) -> (junction 361)
        BackCheck -> (junction 361) [order 1]
        (junction 361) -> (junction 362) [order 1] : /* 靠背不满足角度需求 */
            | [BackMoreThanFlg == FALSE]
        (junction 361) -> (junction 363) [order 2]
        (junction 362) -> (junction 373) : {WelcomeBackReqPosi = BackMoreThanHall;
            | WelcomeReqCMD = TRUE;}
        (junction 373) -> (junction 363)
        (junction 363) -> (junction 367) : {WelcomeRunStatus = 14;}
      state BackwardSuccess
        en:
        /*迎宾默认状态：1.舒适请求 = 无；
        2.迎宾坐标 = 0；*/
        WelcomeReqCMD = FALSE;
        WelcomeReqPosi = 0;
        WelcomeBackReqPosi = 0;
        WelcomeRunStatus = ...
        enWelcomeRunSts.EN_Wel_BWMoveSuccess;
      state BackwardRunning
        en:
        WelcomeBackReqPosi = 0;
        WelcomeStatus = enWelcomeSts.EN_Wel_BWOngoing;
        WelcomeRunStatus = enWelcomeRunSts.EN_Wel_BWOngoing
        WelcomeReqCMD = TRUE;
        WelcomeReqPosi = LocalLengthReqPosi;
        du:
        WelcomeReqPosi = LocalLengthReqPosi;
      (default) -> BackCheck
      WelcomeBackward -> (junction 325) [order 1]
      (junction 325) -> (junction 326) [order 1] : /*有默认状态进入&& (EEPROM要求更新迎宾坐标 || 坐标数据异常) */
          | [TRUE == WelcomeFromeInitFlag ...
          | && (TRUE == MtrWel_UpdatePosiFlag ...
          | || MtrWel_LengthBWTargetPosi == 0 || MtrWel_LengthBWTargetPosi == 0xFFFF ...
          | || MtrWel_LengthFWTargetPosi == 0 || MtrWel_LengthFWTargetPosi == 0xFFFF ...
          | || MtrWel_LengthFWTargetPosi < MtrWel_LengthBWTargetPosi)]
      (junction 325) -> (junction 329) [order 2] : {LocalLengthReqPosi = MtrWel_LengthBWTargetPosi;}
      (junction 326) -> (junction 327) : {/*清初始化跳转标志位、清更新迎宾坐标标志位、更新前移坐标*/
          | WelcomeFromeInitFlag = FALSE;
          | TempPosi = MtrWel_LengthHallPosi - D_WelcomeDistance;
          | Set_WelcomeUpdatePosiFlag(FALSE);
          | Set_WelcomeFWTargertPosi(MtrWel_LengthHallPosi);}
      (junction 327) -> (junction 328) [order 1] : /*后移目标位置是否超过软止点*/
          | [TempPosi > (MtrWel_LengthStopPosi + D_SoftDistancePaLegnth)]
      (junction 327) -> (junction 330) [order 2] : {LocalLengthReqPosi = MtrWel_LengthStopPosi + D_SoftDistancePaLegnth;}
      (junction 328) -> (junction 331) : {LocalLengthReqPosi = TempPosi;}
      BackCheck -> BackwardRunning [order 1] : /* 靠背满足角度需求 */
          | [BackMoreThanFlg == TRUE]
      (junction 331) -> (junction 330)
      (junction 330) -> (junction 381) : {/*存储后移目标坐标*/
          | Set_WelcomeBWTargertPosi(LocalLengthReqPosi);}
      (junction 381) -> (junction 329)
      (junction 329) -> (junction 332)
      BackwardRunning -> BackwardSuccess : /*运行到后移目标位置*/
          | [enSeatAutoRunSts.EN_SEAT_SUCCESS == MtrWel_LengthAutoRunFlag]
          | /WelcomeStatus = enWelcomeSts.EN_BackwardStsSuccess;
          | WelcomeRunStatus = enWelcomeRunSts.EN_Wel_BWMoveSuccess;
          | Set_WelcomeStatus(WelcomeStatus);
    state WelcomeForward
      en:
      /*迎宾状态 = 前移*/
      /*防止突然掉电后下次不能在执行后移*/
      WelcomeStatus = enWelcomeSts.EN_Wel_FWOngoing;
      Set_WelcomeStatus(WelcomeStatus);
      /*迎宾前移：
      1.运行状态 = 前移运行中；
      2.舒适请求 = 前移；
      3.迎宾坐标 = 前移目标坐标；*/
      WelcomeRunStatus = enWelcomeRunSts.EN_Wel_FWOngoing;
      WelcomeReqCMD = TRUE;
      WelcomeReqPosi = MtrWel_LengthFWTargetPosi;
      WelcomeBackReqPosi = 0;
    (default) -> WelcomeDefault
    WelcomeDefault -> WelcomeBackward [order 1] : /*满足后移条件&&上一次未成功执行后移*/
        | [hasChangedTo(BackwardTriggerCondition,TRUE) ...
        | && enWelcomeSts.EN_BackwardStsSuccess != WelcomeStatus]
        | /WelcomeFromeInitFlag = TRUE;
    WelcomeDefault -> BackwardSuccess [order 2] : /*后移成功&&没有打断过（增加原因mantis：7341）*/
        | [enWelcomeSts.EN_BackwardStsSuccess == WelcomeStatus ...
        | && MtrWel_UpdatePosiFlag == FALSE]
    WelcomeForward -> WelcomeDefault [order 2] : /*运动到目标坐标*/
        | [enSeatAutoRunSts.EN_SEAT_SUCCESS == MtrWel_LengthAutoRunFlag]
        | /WelcomeRunStatus = enWelcomeRunSts.EN_Wel_FWMoveSuccess;
        | WelcomeStatus = enWelcomeSts.EN_ForwardStsSuccess;
        | Set_WelcomeStatus(WelcomeStatus);
    WelcomeBackward -> WelcomeForward [order 1] : /*满足前移条件*/
        | [hasChangedTo(ForwardTriggerCondition,TRUE)]
        | //WelcomeStatus = enWelcomeSts.EN_BackMovingExForWard
    WelcomeForward -> WelcomeBackward [order 1] : /*满足后移条件*/
        | [hasChangedTo(BackwardTriggerCondition,TRUE)]
        | //WelcomeStatus = enWelcomeSts.EN_ForWardMovingExBack
  (default) -> Init
  WelcomeInactive -> WelcomeActive [order 1] : /*迎宾前置条件满足*/
      | [enWelStopCause.EN_WelStop_NULL == WelcomeStopReason]
      | /WelcomeRunStatus = 11;
  WelcomeActive -> WelcomeInactive [order 1] : /*前移过程中||后移过程中前置条件不满足，下次需要更新目标坐标*/
      | [(WelcomeStatus == enWelcomeSts.EN_Wel_FWOngoing ...
      | || WelcomeStatus == enWelcomeSts.EN_Wel_BWOngoing) ...
      | && enWelStopCause.EN_WelStop_NULL != WelcomeStopReason]
      | /WelcomeStopReasonOut = WelcomeStopReason;
      | Set_WelcomeUpdatePosiFlag(TRUE);
  WelcomeActive -> WelcomeInactive [order 2] : /*存在纵向霍尔故障*/
      | [TRUE == MtrWel_LengthHallFaultSts]
      | /WelcomeStopReasonOut = enWelStopCause.EN_WelStop_HallFault;
      | Set_WelcomeUpdatePosiFlag(TRUE);
  WelcomeActive -> WelcomeInactive [order 4] : /* 靠背霍尔故障*/
      | [TRUE == MtrWel_BackHallFaultSts]
      | /WelcomeStopReasonOut = enWelStopCause.EN_WelStop_HallFault;
  WelcomeActive -> WelcomeInactive [order 3] : /*前置条件不满足，且不需要更新目标坐标*/
      | [enWelStopCause.EN_WelStop_NULL != WelcomeStopReason]
      | /WelcomeStopReasonOut = WelcomeStopReason;
  Init -> WelcomeActive : /*初始化完成，获取迎宾状态*/
      | [InitTimer > D_InitDelayTime]
      | /WelcomeStatus = MtrWel_WelcomeStatus;
      | WelcomeRunStatus = 13;
  data: In1 function_input; In1 function_input; In1 function_input; In1 function_input; BackwardTriggerCondition input; ForwardTriggerCondition input; WelcomeStopReason input; MtrWel_LengthHallFaultSts input; MtrWel_LengthStopPosi input; MtrWel_LengthHallPosi input; MtrWel_LengthFWTargetPosi input; MtrWel_LengthBWTargetPosi input; MtrWel_LengthAutoRunFlag input; TRUE parameter; FALSE parameter; MtrWel_WelcomeStatus input; D_WelcomeDistance parameter; D_SoftDistancePaLegnth parameter; TempPosi local uint16; WelcomeFromeInitFlag local uint8; WelcomeStopReasonOut output uint8; WelcomeStatus local Enum: enWelcomeSts; WelcomeRunStatus output uint8; WelcomeReqCMD output uint8; WelcomeReqPosi output uint16; InitTimer local uint8; D_InitDelayTime parameter; MtrWel_UpdatePosiFlag input; MtrWel_BackHallFaultSts input; BackMoreThanFlg input; BackMoreThanHall input; WelcomeBackReqPosi output uint16; LocalLengthReqPosi local uint16

== stateflow chart Appl_PaComfort_CtrlModel/UpDataInputInfo/InputSignalProcess/WelcomePrecondition/Precondition ==
  state CommonCondition [parallel]
    settings: executionOrder=1
    state CommonInit
      en:
      CommonFlag = FALSE;
      WelcomeStopReason = ...
      enWelStopCause.EN_WelStop_VoltageError;
    state CommonActive
      en:
      CommonFlag = TRUE;
    state CommonInactive
      en:
      CommonFlag = FALSE;
    (default) -> CommonInit
    CommonInit -> CommonActive [order 1] : /*迎宾使能 && 无纵向堵转故障 && 无纵向继电器粘连故障
        | && 无靠背堵转故障 && 无靠背继电器粘连故障 && 无busoff故障
        | && 座椅纵向已学习 &&无高优先级运动 && 电压正常*//*&& TRUE == Gear_PN_Flag ...*/
        | [TRUE == ComfortOpenFlag ...
        | && FALSE == MtrWel_LengthLockSts ...
        | && FALSE == MtrWel_LengthRelayFaultSts ...
        | && FALSE == MtrPAWel_BackLockSts ...
        | && FALSE == MtrPAWel_BackRelayFaultSts ...
        | && FALSE == MtrWel_BusoffFlag ...
        | && TRUE == SeatLearnResult ...
        | && enSeatMotorRunType.EN_ComfortEnable >= MtrWel_CurrentMoveType ...
        | && FALSE == MtrWel_0x28E_BDCLostFlag ...
        | && enFinalPowerMode.EN_NORMAL_VOLT == MtrWel_VoltMode ...
        | && TRUE == MtrWel_VoltSatisfy]
        | /WelcomeStopReason = enWelStopCause.EN_WelStop_NULL;
    CommonInactive -> CommonActive : /*迎宾使能 && 无纵向堵转故障 && 无纵向继电器粘连故障
        | && 无靠背堵转故障 && 无靠背继电器粘连故障&& 无busoff故障
        | && 座椅纵向已学习 &&无高优先级运动 && 电压正常*//*&& TRUE == Gear_PN_Flag ...*/
        | [TRUE == ComfortOpenFlag ...
        | && FALSE == MtrWel_LengthLockSts ...
        | && FALSE == MtrWel_LengthRelayFaultSts ...
        | && FALSE == MtrPAWel_BackLockSts ...
        | && FALSE == MtrPAWel_BackRelayFaultSts ...
        | && FALSE == MtrWel_BusoffFlag ...
        | && TRUE == SeatLearnResult ...
        | && enSeatMotorRunType.EN_ComfortEnable >= MtrWel_CurrentMoveType ...
        | && FALSE == MtrWel_0x28E_BDCLostFlag ...
        | && enFinalPowerMode.EN_NORMAL_VOLT == MtrWel_VoltMode ...
        | && TRUE == MtrWel_VoltSatisfy]
        | /WelcomeStopReason = enWelStopCause.EN_WelStop_NULL;
    CommonInit -> CommonInactive [order 2] : /*迎宾禁能*/
        | [TRUE != ComfortOpenFlag]
        | /WelcomeStopReason = enWelStopCause.EN_WelStop_PRM;
        | //Set_WelcomeUpdatePosiFlag(TRUE);
    CommonActive -> CommonInactive [order 1] : /*迎宾禁能*/
        | [TRUE != ComfortOpenFlag]
        | /WelcomeStopReason = enWelStopCause.EN_WelStop_PRM;
        | Set_WelcomeUpdatePosiFlag(TRUE);
    CommonInit -> CommonInactive [commented out] : /*有纵向霍尔故障*/
        | [FALSE != MtrWel_LengthHallFaultSts]
        | /WelcomeStopReason = enWelStopCause.EN_WelStop_HallFault
    CommonActive -> CommonInactive [commented out] : /*有纵向霍尔故障*/
        | [FALSE != MtrWel_LengthHallFaultSts]
        | /WelcomeStopReason = enWelStopCause.EN_WelStop_HallFault
    CommonInit -> CommonInactive [order 3] : /*有纵向或靠背堵转故障*/
        | [FALSE != MtrWel_LengthLockSts || FALSE != MtrPAWel_BackLockSts]
        | /WelcomeStopReason = enWelStopCause.EN_WelStop_LockFault;
        | //Set_WelcomeUpdatePosiFlag(TRUE);
    CommonActive -> CommonInactive [order 2] : /*有纵向或靠背堵转故障*/
        | [FALSE != MtrWel_LengthLockSts || FALSE != MtrPAWel_BackLockSts]
        | /WelcomeStopReason = enWelStopCause.EN_WelStop_LockFault;
        | Set_WelcomeUpdatePosiFlag(TRUE);
    CommonInit -> CommonInactive [order 4] : /*存在纵向或靠背继电器故障*/
        | [FALSE != MtrWel_LengthRelayFaultSts || FALSE != MtrPAWel_BackRelayFaultSts]
        | /WelcomeStopReason = enWelStopCause.EN_WelStop_RelayFault
    CommonActive -> CommonInactive [order 3] : /*存在纵向或靠背继电器故障*/
        | [FALSE != MtrWel_LengthRelayFaultSts  || FALSE != MtrPAWel_BackRelayFaultSts]
        | /WelcomeStopReason = enWelStopCause.EN_WelStop_RelayFault
    CommonInit -> CommonInactive [order 5] : /*有busoff故障*/
        | [FALSE != MtrWel_BusoffFlag]
        | /WelcomeStopReason = enWelStopCause.EN_WelStop_Busoff
    CommonActive -> CommonInactive [order 4] : /*有busoff故障*/
        | [FALSE != MtrWel_BusoffFlag]
        | /WelcomeStopReason = enWelStopCause.EN_WelStop_Busoff
    CommonInit -> CommonInactive [commented out] : /*非PN档*/
        | [TRUE != Gear_PN_Flag]
        | /WelcomeStopReason = enWelStopCause.EN_WelStop_enNotGearPN
    CommonActive -> CommonInactive [commented out] : /*非PN档*/
        | [TRUE != Gear_PN_Flag]
        | /WelcomeStopReason = enWelStopCause.EN_WelStop_enNotGearPN
    CommonInit -> CommonInactive [order 6] : /*纵向、靠背未学习*/
        | [TRUE != SeatLearnResult]
        | /WelcomeStopReason = enWelStopCause.EN_WelStop_enNotLearn;
        | //Set_WelcomeUpdatePosiFlag(TRUE);
    CommonActive -> CommonInactive [order 5] : /*纵向、靠背未学习*/
        | [TRUE != SeatLearnResult]
        | /WelcomeStopReason = enWelStopCause.EN_WelStop_enNotLearn;
        | Set_WelcomeUpdatePosiFlag(TRUE);
    CommonInit -> CommonInactive [order 7] : /*有高由于迎宾运动的请求*/
        | [enSeatMotorRunType.EN_ComfortEnable < MtrWel_CurrentMoveType]
        | /WelcomeStopReason = enWelStopCause.EN_WelStop_OtherMove;
        | //Set_WelcomeUpdatePosiFlag(TRUE);
    CommonActive -> CommonInactive [order 6] : /*有高由于迎宾运动的请求*/
        | [enSeatMotorRunType.EN_ComfortEnable < MtrWel_CurrentMoveType]
        | /WelcomeStopReason = enWelStopCause.EN_WelStop_OtherMove;
        | Set_WelcomeUpdatePosiFlag(TRUE);
    CommonInit -> CommonInactive [order 8] : /*门信号丢失*/
        | [TRUE == MtrWel_0x28E_BDCLostFlag]
        | /WelcomeStopReason = enWelStopCause.EN_WelStop_enBDCDoorLost
    CommonActive -> CommonInactive [order 7] : /*门信号丢失*/
        | [TRUE == MtrWel_0x28E_BDCLostFlag]
        | /WelcomeStopReason = enWelStopCause.EN_WelStop_enBDCDoorLost
    CommonInit -> CommonInactive [order 9] : /*电压非正常模式*/
        | [enFinalPowerMode.EN_NORMAL_VOLT != MtrWel_VoltMode ...
        | || TRUE != MtrWel_VoltSatisfy]
        | /WelcomeStopReason = enWelStopCause.EN_WelStop_VoltageError
    CommonActive -> CommonInactive [order 8] : /*电压非正常模式*/
        | [enFinalPowerMode.EN_NORMAL_VOLT != MtrWel_VoltMode ...
        | || TRUE != MtrWel_VoltSatisfy]
        | /WelcomeStopReason = enWelStopCause.EN_WelStop_VoltageError
  state Set_WelcomeUpdatePosiFlag(In1) [function]
  state DoorSts [parallel]
    settings: executionOrder=2
    state DoorInit
      en:
      WaitTimeCnt = 0;
      LocalDoorSts = 0xFF;
      du:
      WaitTimeCnt += 1;
      LocalDoorSts = Get_DoorSts();
      ex:
      WaitTimeCnt = 0;
      LocalDoorSts = Get_DoorSts();
    state DoorSts1
      du:
      LocalDoorSts = MtrWel_BDC_FRDoorSts;
      E2pDoorSts = Get_DoorSts();
      state BackwardTriggerCondition [parallel]
        settings: executionOrder=1
        state BWActive
          en:
          BackwardTriggerCondition = TRUE;
        state BWInactive
          en:
          BackwardTriggerCondition = FALSE;
        (default) -> BWInactive
        BWInactive -> BWActive : /* 迎宾后移条件
            | C5、右前车门状态由关闭→打开（BDC_FRDoorSts=0x0:Close→0x1:Open）且前数据正常*/
            | [hasChangedTo(LocalDoorSts,D_OPEN) ...
            | && E2pDoorSts <= D_OPEN]
        BWActive -> BWInactive : /*2个运行周期*/
            | after(2,tick)
      state Change [parallel]
        settings: executionOrder=3
        Change -> (junction 214)
        (junction 214) -> (junction 225)
        (junction 225) -> (junction 216) [order 1] : /* 门状态变化 存数据 */
            | [hasChanged(LocalDoorSts) && LocalDoorSts <= D_OPEN]
        (junction 225) -> (junction 222) [order 2]
        (junction 216) -> (junction 219) : {Set_DoorSts(LocalDoorSts);}
        (junction 219) -> (junction 222)
        (junction 222) -> (junction 221)
      state ForwardTriggercondition [parallel]
        settings: executionOrder=2
        state FWInactive
          en:
          ForwardTriggerCondition = FALSE;
        state FWActive
          en:
          ForwardTriggerCondition = TRUE;
        (default) -> FWInactive
        FWInactive -> FWActive : /* 迎宾前移条件
            | C6、右前车门状态由打开→关闭（BDC_FRDoorSts=0x1:Open→0x0:Close）且前数据正常*/
            | [hasChangedTo(LocalDoorSts,D_CLOSE)...
            | && E2pDoorSts <= D_OPEN]
        FWActive -> FWInactive : /*2个运行周期*/
            | after(2,tick)
    (default) -> DoorInit
    DoorInit -> DoorSts1 : /* 等待读取e2p数据 */
        | [WaitTimeCnt > 20]
  state Set_DoorSts(In1) [function]
  state UpdatePosi [parallel]
    settings: executionOrder=3
    (default) -> (junction 246)
    UpdatePosi -> (junction 246)
    (junction 246) -> (junction 239)
    (junction 239) -> (junction 243) [order 1] : /* 纵向坐标变化 且非舒适功能调节 需要更新纵向位置 */
        | [enSeatMotorRunType.EN_ComfortEnable != MtrWel_CurrentMoveType ...
        | && enSeatMotorRunType.EN_NULL != MtrWel_CurrentMoveType ...
        | && (hasChangedTo(MtrPAWel_LengthCmd,1) || hasChangedTo(MtrPAWel_LengthCmd,2))]
    (junction 239) -> (junction 237) [order 2]
    (junction 243) -> (junction 235) : {Set_WelcomeUpdatePosiFlag(TRUE);}
    (junction 235) -> (junction 237)
    (junction 237) -> (junction 236)
  state Out1 = Get_DoorSts [function]
  data: In1 function_input; In1 function_input; Out1 function_output; ComfortOpenFlag input; Gear_PN_Flag input; MtrWel_LengthLockSts input; MtrWel_BusoffFlag input; CommonFlag local uint8; FALSE parameter; TRUE parameter; BackwardTriggerCondition output uint8; ForwardTriggerCondition output uint8; WelcomeStopReason output Enum: enWelStopCause =enWelStopCause.EN_WelStop_VoltageError; MtrWel_CurrentMoveType input; SeatLearnResult input; MtrWel_LengthRelayFaultSts input; MtrWel_0x28E_BDCLostFlag input; MtrWel_BDC_FRDoorSts input; D_OPEN parameter; D_CLOSE parameter; MtrWel_VoltMode input; MtrWel_VoltSatisfy input; MtrPAWel_BackHallFaultSts input; MtrPAWel_BackRelayFaultSts input; MtrPAWel_BackLockSts input; LocalDoorSts local uint8; WaitTimeCnt local uint8; MtrPAWel_LengthCmd input; E2pDoorSts local uint8
